simulink model "pf_ca2_02_03"  (R2023b)
settings: Solver=VariableStepAuto  StartTime=0.0  StopTime=15  RelTol=1e-3
settings Model: Creator=stem  LastModifiedBy=stem

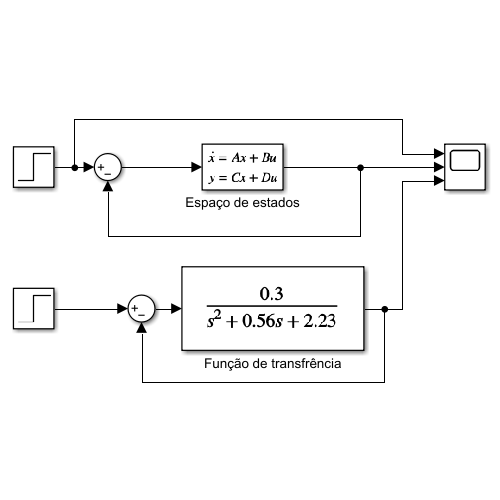
[thumbnail: Simulink's stored preview of the top-level diagram]
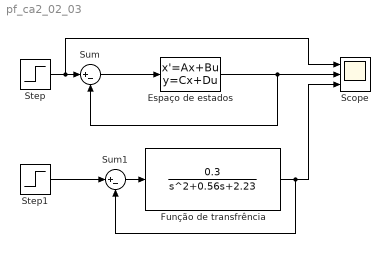
== system pf_ca2_02_03 ==
  Espaço de estados : StateSpace  A=[0 1 ; -2.23 -0.56]  B=[0 ; 0.3]  C=[1 0]  D=0  InitialCondition=0
  Função de transfrência : TransferFcn  Numerator=[0.3]  Denominator=[1 0.56 2.23]
  Scope : Scope  NumInputPorts=3
  Step : Step  After=100  SampleTime=0
  Step1 : Step  After=100  SampleTime=0
  Sum : Sum  Inputs=|+-
  Sum1 : Sum  Inputs=|+-
  wires:
  Espaço de estados/1 -> Sum/2, Scope/2
  Sum/1 -> Espaço de estados/1
  Step/1 -> Scope/1, Sum/1
  Step1/1 -> Sum1/1
  Sum1/1 -> Função de transfrência/1
  Função de transfrência/1 -> Scope/3, Sum1/2
